simulink model "spm2"  (Simulink 3.00)
settings: Solver=ode45  SolverMode=SingleTasking  StartTime=0.0  StopTime=999999  MaxStep=10  RelTol=1e-3  AbsTol=1e-6
settings Model: SaveTime=off  SaveOutput=off

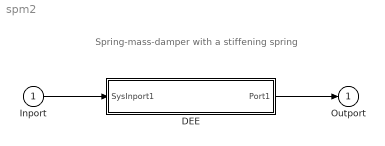
== system spm2 ==
  note: Spring-mass-damper with a stiffening spring
  Inport : Inport  Port=1  PortWidth=-1  SampleTime=-1  DataType=auto
      settings: SignalType=auto
  DEE : Subsystem
      settings: OpenFcn=diffeqed
      mask Type: Differential Equation Editor (DEE)
      mask Display: disp('Spring-mass-damper\nsystem')
  Outport : Outport  Port=1
  wires:
  Inport/1 -> DEE/1(SysInport1)
  DEE/1(Port1) -> Outport/1

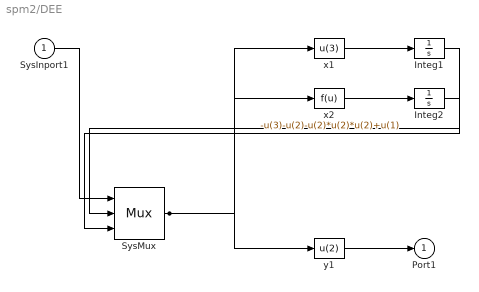
== system spm2/DEE ==
  SysInport1 : Inport  Port=1  PortWidth=-1  SampleTime=-1  DataType=auto
      settings: SignalType=auto
  Integ1 : Integrator  ExternalReset=none  InitialConditionSource=internal  InitialCondition=0  LimitOutput=off  UpperSaturationLimit=inf  LowerSaturationLimit=-inf  ShowSaturationPort=off  ShowStatePort=off  AbsoluteTolerance=auto
  Integ2 : Integrator  ExternalReset=none  InitialConditionSource=internal  InitialCondition=0  LimitOutput=off  UpperSaturationLimit=inf  LowerSaturationLimit=-inf  ShowSaturationPort=off  ShowStatePort=off  AbsoluteTolerance=auto
  SysMux : Mux  Inputs=3
      settings: DisplayOption=none
  x1 : Fcn  Expr=u(3)
  x2 : Fcn  Expr=-u(3)-u(2)-u(2)*u(2)*u(2)+u(1)
  y1 : Fcn  Expr=u(2)
  Port1 : Outport  Port=1
  wires:
  y1/1 -> Port1/1
  Integ2/1 -> SysMux/3
  x2/1 -> Integ2/1
  SysMux/1 -> y1/1, x2/1, x1/1
  Integ1/1 -> SysMux/2
  x1/1 -> Integ1/1
  SysInport1/1 -> SysMux/1
